simulink model "TST_ASDdc_SelectParameter"  (R2016b)
settings: Solver=FixedStepDiscrete  StartTime=0.0  StopTime=simTime  FixedStep=sampleTime  RelTol=1e-3
values from neighbouring files (symbols this model uses):
  testCase = 1    [initTST_ASDdc_SelectParameter_001.m]
libraries: simulink x2
settings Model: Creator=lenovo  LastModifiedBy=lenovo
settings DebuggingCC: SignalRangeChecking=error

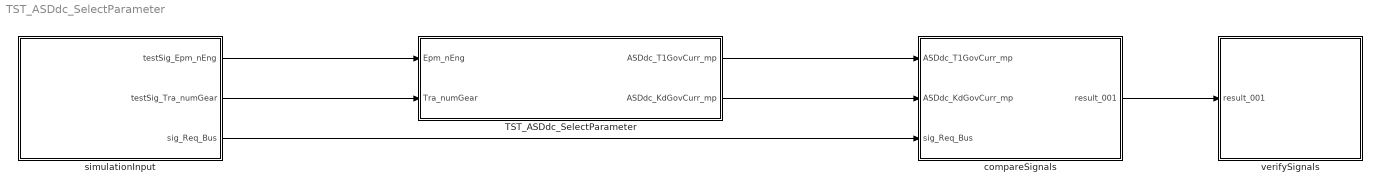
== system TST_ASDdc_SelectParameter ==
  TST_ASDdc_SelectParameter : Subsystem
  compareSignals : Subsystem
  simulationInput : Subsystem
  verifySignals : Subsystem
  wires:
  simulationInput/1(testSig_Epm_nEng) -> TST_ASDdc_SelectParameter/1(Epm_nEng)
  simulationInput/2(testSig_Tra_numGear) -> TST_ASDdc_SelectParameter/2(Tra_numGear)
  TST_ASDdc_SelectParameter/1(ASDdc_T1GovCurr_mp) -> compareSignals/1(ASDdc_T1GovCurr_mp)
  TST_ASDdc_SelectParameter/2(ASDdc_KdGovCurr_mp) -> compareSignals/2(ASDdc_KdGovCurr_mp)
  simulationInput/3(sig_Req_Bus) -> compareSignals/3(sig_Req_Bus)
  compareSignals/1(result_001) -> verifySignals/1(result_001)

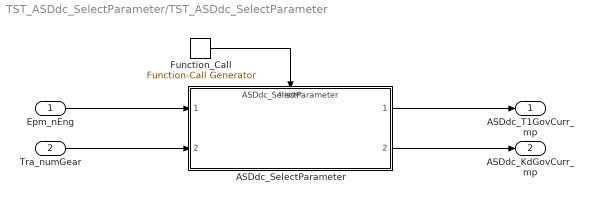
== system TST_ASDdc_SelectParameter/TST_ASDdc_SelectParameter ==
  Epm_nEng : Inport
  Tra_numGear : Inport  Port=2
  ASDdc_SelectParameter : ModelReference  ModelNameDialog=ASDdc_SelectParameter  ModelReferenceVersion=1.24  TriggerPortName=function  TriggerPortTriggerType=function-call  TriggerPortStatesWhenEnabling=held
  Function_Call : simulink/Ports & Subsystems/Function-Call Generator  sample_time=sampleTime  numberOfIterations=1
  ASDdc_T1GovCurr_mp : Outport
  ASDdc_KdGovCurr_mp : Outport  Port=2
  wires:
  Function_Call/1 -> ASDdc_SelectParameter/Trigger
  Epm_nEng/1 -> ASDdc_SelectParameter/1
  Tra_numGear/1 -> ASDdc_SelectParameter/2
  ASDdc_SelectParameter/1 -> ASDdc_T1GovCurr_mp/1
  ASDdc_SelectParameter/2 -> ASDdc_KdGovCurr_mp/1

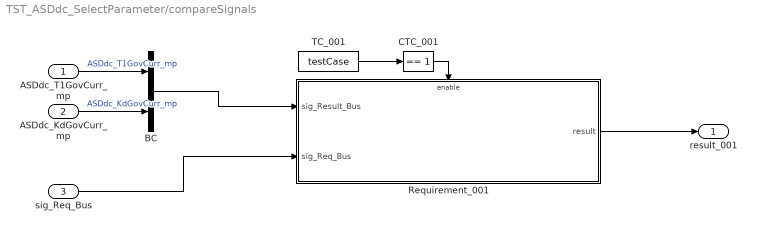
== system TST_ASDdc_SelectParameter/compareSignals ==
  ASDdc_T1GovCurr_mp : Inport
  ASDdc_KdGovCurr_mp : Inport  Port=2
  sig_Req_Bus : Inport  Port=3
  BC : BusCreator  Inputs=2
  CTC_001 : simulink/Logic and Bit Operations/Compare To Constant  relop===  const=1  OutDataTypeStr=boolean
  Requirement_001 : Subsystem
  TC_001 : Constant  Value=testCase
  result_001 : Outport
  wires:
  ASDdc_T1GovCurr_mp/1 -> BC/1  "ASDdc_T1GovCurr_mp"
  ASDdc_KdGovCurr_mp/1 -> BC/2  "ASDdc_KdGovCurr_mp"
  TC_001/1 -> CTC_001/1
  CTC_001/1 -> Requirement_001/Enable
  sig_Req_Bus/1 -> Requirement_001/2(sig_Req_Bus)
  BC/1 -> Requirement_001/1(sig_Result_Bus)
  Requirement_001/1(result) -> result_001/1

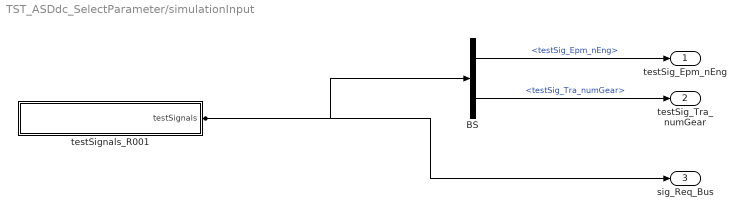
== system TST_ASDdc_SelectParameter/simulationInput ==
  BS : BusSelector  OutputSignals=testSig_Epm_nEng,testSig_Tra_numGear
  testSignals_R001 : Subsystem
  testSig_Epm_nEng : Outport
  testSig_Tra_numGear : Outport  Port=2
  sig_Req_Bus : Outport  Port=3
  wires:
  BS/1 -> testSig_Epm_nEng/1  "<testSig_Epm_nEng>"
  BS/2 -> testSig_Tra_numGear/1  "<testSig_Tra_numGear>"
  testSignals_R001/1(testSignals) -> BS/1, sig_Req_Bus/1

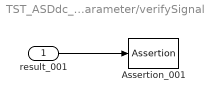
== system TST_ASDdc_SelectParameter/verifySignals ==
  result_001 : Inport
  Assertion_001 : Assertion
  wires:
  result_001/1 -> Assertion_001/1

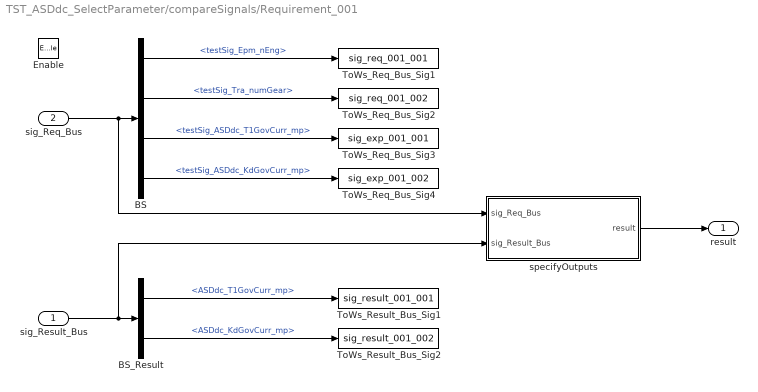
== system TST_ASDdc_SelectParameter/compareSignals/Requirement_001 ==
  sig_Result_Bus : Inport
  sig_Req_Bus : Inport  Port=2
  Enable : EnablePort
  BS : BusSelector  OutputSignals=testSig_Epm_nEng,testSig_Tra_numGear,testSig_ASDdc_T1GovCurr_mp,testSig_ASDdc_KdGovCurr_mp
  BS_Result : BusSelector  OutputSignals=ASDdc_T1GovCurr_mp,ASDdc_KdGovCurr_mp
  ToWs_Req_Bus_Sig1 : ToWorkspace  VariableName=sig_req_001_001  SaveFormat=Structure With Time
  ToWs_Req_Bus_Sig2 : ToWorkspace  VariableName=sig_req_001_002  SaveFormat=Structure With Time
  ToWs_Req_Bus_Sig3 : ToWorkspace  VariableName=sig_exp_001_001  SaveFormat=Structure With Time
  ToWs_Req_Bus_Sig4 : ToWorkspace  VariableName=sig_exp_001_002  SaveFormat=Structure With Time
  ToWs_Result_Bus_Sig1 : ToWorkspace  VariableName=sig_result_001_001  SaveFormat=Structure With Time
  ToWs_Result_Bus_Sig2 : ToWorkspace  VariableName=sig_result_001_002  SaveFormat=Structure With Time
  specifyOutputs : Subsystem
  result : Outport
  wires:
  sig_Req_Bus/1 -> BS/1, specifyOutputs/1(sig_Req_Bus)
  BS/1 -> ToWs_Req_Bus_Sig1/1  "<testSig_Epm_nEng>"
  BS/2 -> ToWs_Req_Bus_Sig2/1  "<testSig_Tra_numGear>"
  BS/3 -> ToWs_Req_Bus_Sig3/1  "<testSig_ASDdc_T1GovCurr_mp>"
  BS/4 -> ToWs_Req_Bus_Sig4/1  "<testSig_ASDdc_KdGovCurr_mp>"
  sig_Result_Bus/1 -> BS_Result/1, specifyOutputs/2(sig_Result_Bus)
  BS_Result/1 -> ToWs_Result_Bus_Sig1/1  "<ASDdc_T1GovCurr_mp>"
  BS_Result/2 -> ToWs_Result_Bus_Sig2/1  "<ASDdc_KdGovCurr_mp>"
  specifyOutputs/1(result) -> result/1

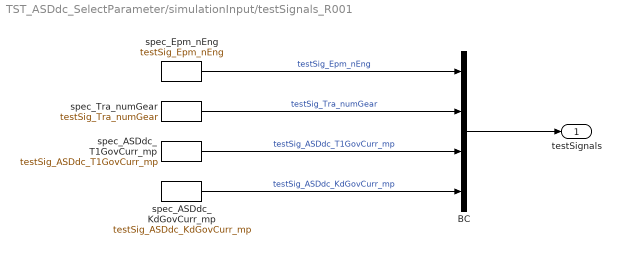
== system TST_ASDdc_SelectParameter/simulationInput/testSignals_R001 ==
  BC : BusCreator  Inputs=4
  spec_ASDdc_KdGovCurr_mp : FromWorkspace  VariableName=testSig_ASDdc_KdGovCurr_mp  Interpolate=off  OutputAfterFinalValue=Holding final value
  spec_ASDdc_T1GovCurr_mp : FromWorkspace  VariableName=testSig_ASDdc_T1GovCurr_mp  Interpolate=off  OutputAfterFinalValue=Holding final value
  spec_Epm_nEng : FromWorkspace  VariableName=testSig_Epm_nEng  Interpolate=off  OutputAfterFinalValue=Holding final value
  spec_Tra_numGear : FromWorkspace  VariableName=testSig_Tra_numGear  Interpolate=off  OutputAfterFinalValue=Holding final value
  testSignals : Outport
  wires:
  BC/1 -> testSignals/1
  spec_Epm_nEng/1 -> BC/1  "testSig_Epm_nEng"
  spec_Tra_numGear/1 -> BC/2  "testSig_Tra_numGear"
  spec_ASDdc_T1GovCurr_mp/1 -> BC/3  "testSig_ASDdc_T1GovCurr_mp"
  spec_ASDdc_KdGovCurr_mp/1 -> BC/4  "testSig_ASDdc_KdGovCurr_mp"

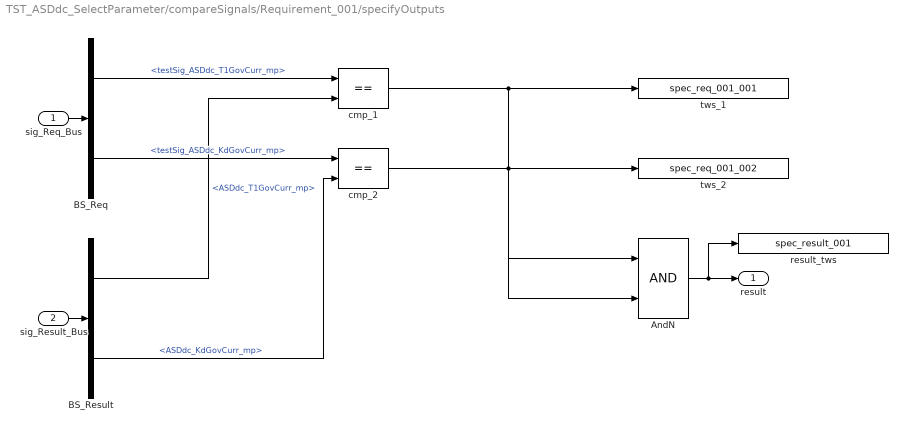
== system TST_ASDdc_SelectParameter/compareSignals/Requirement_001/specifyOutputs ==
  sig_Req_Bus : Inport
  sig_Result_Bus : Inport  Port=2
  AndN : Logic
  BS_Req : BusSelector  OutputSignals=testSig_ASDdc_T1GovCurr_mp,testSig_ASDdc_KdGovCurr_mp
  BS_Result : BusSelector  OutputSignals=ASDdc_T1GovCurr_mp,ASDdc_KdGovCurr_mp
  cmp_1 : RelationalOperator  Operator===  RndMeth=Nearest  InputSameDT=on
  cmp_2 : RelationalOperator  Operator===  RndMeth=Nearest  InputSameDT=on
  result_tws : ToWorkspace  VariableName=spec_result_001
  tws_1 : ToWorkspace  VariableName=spec_req_001_001
  tws_2 : ToWorkspace  VariableName=spec_req_001_002
  result : Outport
  wires:
  sig_Req_Bus/1 -> BS_Req/1
  sig_Result_Bus/1 -> BS_Result/1
  AndN/1 -> result/1, result_tws/1
  BS_Req/1 -> cmp_1/1  "<testSig_ASDdc_T1GovCurr_mp>"
  BS_Result/1 -> cmp_1/2  "<ASDdc_T1GovCurr_mp>"
  cmp_1/1 -> tws_1/1, AndN/1
  BS_Req/2 -> cmp_2/1  "<testSig_ASDdc_KdGovCurr_mp>"
  BS_Result/2 -> cmp_2/2  "<ASDdc_KdGovCurr_mp>"
  cmp_2/1 -> tws_2/1, AndN/2
